simulink model "car"  (R2022a)
settings: Solver=VariableStepAuto  StartTime=0.0  StopTime=10.0  RelTol=1e-3
settings Model: Creator=Taha  LastModifiedBy=Asus
settings SolverCC: AlgebraicLoopSolver=TrustRegion
settings DebuggingCC: UnconnectedInputMsg=warning  UnconnectedOutputMsg=warning  UnconnectedLineMsg=warning  SFMachineParentedDataDiag=warning
settings RTWCC: DLArmComputeVersion=19.05

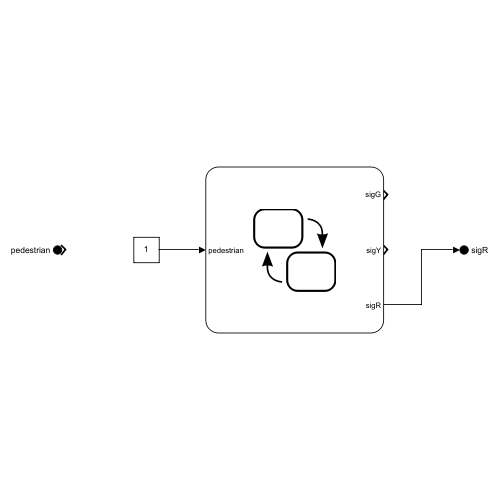
[thumbnail: Simulink's stored preview of the top-level diagram]
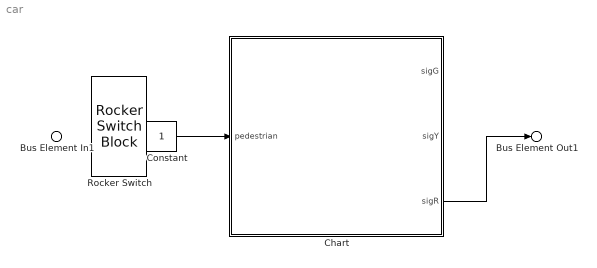
== system car ==
  Bus Element In1 : Inport  PortName=pedestrian
  Chart : Stateflow chart  TreatAsAtomicUnit=on
      settings: PortSchema="{\"entries\":[{\"content\":{\"sides\":[{\"content\":{\"connectorIds\":[\"In1\"]},\"type\":\"ConnectorPlacement.EquallySpacedRectSide\",\"uuid\":\"0472c1e1-a4ac-46d8-983b-419c5abeaf89\"},{\"content\":{\"connectorIds\":[\"Out3\",\"Out1\",\"Out2\"],\"side\":\"RIGHT\"},\"type\":\"ConnectorPlacement.EquallySpacedRectSide\",\"uuid\":\"25d0bf68-89c1-4ea6-8460-438ed2268ffb\"},{\"content\":{\"connectorIds\":[],\"side\":\"TOP\"},\"type\":\"ConnectorPlacement.EquallySpacedRectSide\",\"uuid\":\"acb93bac-ff43-46d0-a81c-cac848a50315\"}]},\"type\":\"ConnectorPlacement.EquallySpacedConnector\",\"uuid\":\"5c7cc856-7ee7-4b66-af73-db569f5542a8\"}],\"packageUris\":[\"http://schema.mathworks.com/mf0/Connector/R2020b\"],\"version\":\"1.0\"}"
  Constant : Constant
  Rocker Switch : RockerSwitchBlock
      settings: Values={{'Off', 'On'}, [0 1]}
  Bus Element Out1 : Outport  PortName=sigR
  wires:
  Chart/2(sigR) -> Bus Element Out1/1
  Constant/1 -> Chart/1(pedestrian)

== stateflow chart car/Chart ==
  state green
  state red
  state pending
  state yellow
  green -> green [order 3] : [count<60]
      | {count=count+1;}
  red -> green [order 1] : [count>=60]
      | {sigG=1;count=0;}
  green -> pending [order 1] : [pedestrian==1 && count<60]
      | {count=count+1;}
  green -> yellow [order 2] : [pedestrian==1 && count>=60]
      | {sigY=1;count=0;}
  red -> red [order 2] : {count=count+1;}
  pending -> pending [order 2] : {count=count+1;}
  (default) -> red : {count=0;}
  yellow -> red [order 1] : [count>=5]
      | {sigR=1;count=0;}
  pending -> yellow [order 1] : [count>=60]
      | {sigY=1;count=0;}
  yellow -> yellow [order 2] : {count=count+1;}
  data: pedestrian input; sigY output; sigR output; sigG output; count local
